simulink model "first_3phase_multilevel"  (R2015a)
settings: Solver=ode45  StartTime=0.02  StopTime=0.04  RelTol=1e-3
libraries: powerlib x95, powerlib_meascontrol x50, simulink x48, dspstat3 x2
(part 2 of 2)

== matlab function first_3phase_multilevel/position controller23/MATLAB Function9 ==
  data: u input; c input; y output; t input
function y = fcn(u,c,t)
%#codegen
if t>u
    y = 1;
else
    y = 0;
end
if c <0.02
    y = 0;
end

== matlab function first_3phase_multilevel/MATLAB Function4 ==
  data: u input; A1 output; time input; B1 output
function [A1,B1] = fcn(u,time)
%#codegen
A1 = u*sin(13*2*pi*50*time);
B1 = u*cos(13*2*pi*50*time);
end

== matlab function first_3phase_multilevel/MATLAB Function5 ==
  data: u input; A1 output; time input; B1 output
function [A1,B1] = fcn(u,time)
%#codegen
A1 = u*sin(2*pi*50*time);
B1 = u*cos(2*pi*50*time);
end

== matlab function first_3phase_multilevel/position controller24/MATLAB Function10 ==
  data: u input; y output; t input
function y = fcn(u,t)
%#codegen
if t>u
    y = 1;
else
    y = 0;
end
end

== matlab function first_3phase_multilevel/position controller24/MATLAB Function11 ==
  data: u input; c input; y output; t input
function y = fcn(u,c,t)
%#codegen
if t>u
    y = 1;
else
    y = 0;
end
if c<0.02
    y = 0;
end

== matlab function first_3phase_multilevel/position controller25/MATLAB Function12 ==
  data: u input; y output; t input
function y = fcn(u,t)
%#codegen
if t>u
    y = 1;
else
    y = 0;
end
end

== matlab function first_3phase_multilevel/position controller25/MATLAB Function13 ==
  data: u input; c input; y output; t input
function y = fcn(u,c,t)
%#codegen
if t>u
    y = 1;
else
    y = 0;
end
if c<0.02
    y = 0;
end

== matlab function first_3phase_multilevel/MATLAB Function6 ==
  data: u input; A7 output; time input; B7 output
function [A7,B7] = fcn(u,time)
%#codegen
A7 = u*sin(7*2*pi*50*time);
B7 = u*cos(7*2*pi*50*time);
end

== matlab function first_3phase_multilevel/MATLAB Function7 ==
  data: u input; A11 output; time input; B11 output
function [A11,B11] = fcn(u,time)
%#codegen
A11 = u*sin(11*2*pi*50*time);
B11 = u*cos(11*2*pi*50*time);
end

== matlab function first_3phase_multilevel/MATLAB Function8 ==
  data: u input; A5 output; time input; B5 output
function [A5,B5] = fcn(u,time)
%#codegen
A5 = u*sin(5*2*pi*50*time);
B5 = u*cos(5*2*pi*50*time);
end

== matlab function first_3phase_multilevel/MATLAB Function9 ==
  data: u input; A1 output; time input; B1 output
function [A1,B1] = fcn(u,time)
%#codegen
A1 = u*sin(17*2*pi*50*time);
B1 = u*cos(17*2*pi*50*time);
end

== matlab function first_3phase_multilevel/position controller4/MATLAB Function14 ==
  data: u input; y output; t input
function y = fcn(u,t)
%#codegen
if t>u
    y = 1;
else
    y = 0;
end
end

== matlab function first_3phase_multilevel/position controller4/MATLAB Function15 ==
  data: u input; y output; t input
function y = fcn(u,t)
%#codegen
if t>u
    y = 1;
else
    y = 0;
end
end

== matlab function first_3phase_multilevel/position controller5/MATLAB Function1 ==
  data: u input; y output; t input
function y = fcn(u,t)
%#codegen
if t>u
    y = 1;
else
    y = 0;
end
end

== matlab function first_3phase_multilevel/position controller5/MATLAB Function2 ==
  data: u input; y output; t input
function y = fcn(u,t)
%#codegen
if t>u
    y = 1;
else
    y = 0;
end
end

== matlab function first_3phase_multilevel/position controller6/MATLAB Function14 ==
  data: u input; y output; t input
function y = fcn(u,t)
%#codegen
if t>u
    y = 1;
else
    y = 0;
end
end

== matlab function first_3phase_multilevel/position controller6/MATLAB Function15 ==
  data: u input; y output; t input
function y = fcn(u,t)
%#codegen
if t>u
    y = 1;
else
    y = 0;
end
end
